simulink model "s_VI_Operational_pd_wG_ctrl_14bb"  (Simulink 8.4)
settings: Solver=ode45  SolverMode=SingleTasking  StartTime=0.0  StopTime=10.0  RelTol=1e-3
values from neighbouring files (symbols this model uses):
  Kd = 50    [m_IV_run_pd_wG_control_operational.m]
  Kp = 2500    [m_IV_run_pd_wG_control_operational.m]
settings Model: Creator=a_bad  LastModifiedBy=a_bad  CovMetricSettings=dwe  CovHtmlReporting=off  covSaveCumulativeToWorkspaceVar=off  CovSaveSingleToWorkspaceVar=off  CovExternalEMLEnable=on  CovSFcnEnable=on
settings DataIOCC: LimitDataPoints=off  SaveFormat=StructureWithTime  SignalLoggingSaveFormat=Dataset
settings OptimizationCC: ExpressionDepthLimit=128
settings DebuggingCC: AlgebraicLoopMsg=none  UnderspecifiedInitializationDetection=Simplified  MergeDetectMultiDrivingBlocksExec=error  SolverPrmCheckMsg=none  FcnCallInpInsideContextMsg=EnableAllAsError  FrameProcessingCompatibilityMsg=error  StateNameClashWarn=none  SFUnexpectedBacktrackingDiag=error  SFNoUnconditionalDefaultTransitionDiag=error
settings HardwareCC: ProdBitPerPointer=64  ProdLargestAtomicFloat=Float  ProdIntDivRoundTo=Zero  ProdEndianess=LittleEndian  ProdHWDeviceType=Specified
settings ModelReferenceCC: PropagateSignalLabelsOutOfModel=on
settings GRTTargetCC: TargetLangStandard=C99 (ISO)  GeneratePreprocessorConditionals=Use local settings  CombineOutputUpdateFcns=on  GRTInterface=off

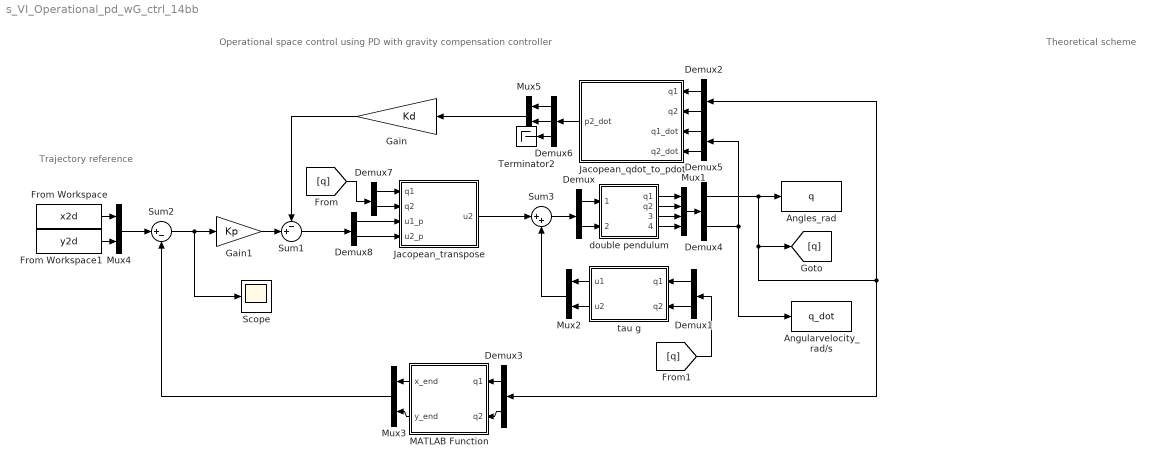
== system s_VI_Operational_pd_wG_ctrl_14bb ==
  note: Theoretical scheme
  note: Trajectory
      | reference
  note: Operational space control using PD with gravity compensation controller
  Angles_rad : ToWorkspace  VariableName=q  SaveFormat=Timeseries  SampleTime=-1
  Angularvelocity_rad/s : ToWorkspace  VariableName=q_dot  SaveFormat=Timeseries  SampleTime=-1
  Demux{,1..5,7..8} (8 alike) : Demux  Outputs=2
  Demux6 : Demux  Outputs=3
  From Workspace : FromWorkspace  VariableName=x2d  SampleTime=0
  From Workspace1 : FromWorkspace  VariableName=y2d  SampleTime=0
  Gain : Gain  Gain=Kd
  Gain1 : Gain  Gain=Kp
  Jacopean_qdot_to_pdot : MATLAB Function  TreatAsAtomicUnit=on
      settings: PermitHierarchicalResolution=ParametersOnly
  Jacopean_transpose : MATLAB Function  TreatAsAtomicUnit=on
      settings: PermitHierarchicalResolution=ParametersOnly
  MATLAB Function : MATLAB Function  TreatAsAtomicUnit=on
      settings: PermitHierarchicalResolution=ParametersOnly
  Mux1 : Mux
  Mux{2..5} (4 alike) : Mux  Inputs=2
  Scope : Scope
      settings: TimeRange=auto  MaxDataPoints=5000  SaveToWorkspace=off  SaveName=ScopeData  YMin=-0.05308  YMax=0.10902  SampleTime=-1
  Sum1 : Sum  Inputs=-+|
  Sum2 : Sum  Inputs=|+-
  Sum3 : Sum  Inputs=|++
  Terminator2 : Terminator
  "double pendulum " : Subsystem
      mask Display: image('294px-Double-Pendulum.svg.png');
  "tau g " : MATLAB Function  TreatAsAtomicUnit=on
      settings: PermitHierarchicalResolution=ParametersOnly
  wires:
  "double pendulum "/1(q1) -> Mux1/1
  Demux/1 -> "double pendulum "/1(Tau1)
  Demux/2 -> "double pendulum "/2("Tau2 ")
  "double pendulum "/4(q2_dot) -> Mux1/4
  "double pendulum "/2("q2  ") -> Mux1/2
  "double pendulum "/3("q1_dot ") -> Mux1/3
  Mux1/1 -> Demux4/1
  Demux4/2 -> Angularvelocity_rad/s/1, Demux5/1
  Demux4/1 -> Demux3/1, Demux2/1, [q], Angles_rad/1
  From Workspace/1 -> Mux4/1
  From Workspace1/1 -> Mux4/2
  Mux4/1 -> Sum2/1
  Demux1/1 -> "tau g "/1(q1)
  Demux1/2 -> "tau g "/2(q2)
  "tau g "/1(u1) -> Mux2/1
  "tau g "/2(u2) -> Mux2/2
  Sum3/1 -> Demux/1
  Demux3/1 -> MATLAB Function/1(q1)
  Demux3/2 -> MATLAB Function/2(q2)
  Mux2/1 -> Sum3/2
  MATLAB Function/1(x_end) -> Mux3/1
  MATLAB Function/2(y_end) -> Mux3/2
  Mux3/1 -> Sum2/2
  Demux2/1 -> Jacopean_qdot_to_pdot/1(q1)
  Demux2/2 -> Jacopean_qdot_to_pdot/2(q2)
  Demux5/1 -> Jacopean_qdot_to_pdot/3(q1_dot)
  Demux5/2 -> Jacopean_qdot_to_pdot/4(q2_dot)
  Jacopean_qdot_to_pdot/1(p2_dot) -> Demux6/1
  Demux6/3 -> Terminator2/1
  Demux6/1 -> Mux5/1
  Demux6/2 -> Mux5/2
  Mux5/1 -> Gain/1
  Sum2/1 -> Scope/1, Gain1/1
  Gain/1 -> Sum1/1
  Gain1/1 -> Sum1/2
  Demux7/1 -> Jacopean_transpose/1(q1)
  Demux7/2 -> Jacopean_transpose/2(q2)
  [q] -> Demux7/1
  Sum1/1 -> Demux8/1
  Demux8/1 -> Jacopean_transpose/3(u1_p)
  Demux8/2 -> Jacopean_transpose/4(u2_p)
  Jacopean_transpose/1(u2) -> Sum3/1
  [q] -> Demux1/1

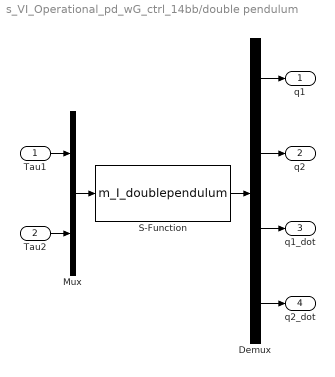
== system s_VI_Operational_pd_wG_ctrl_14bb/double pendulum  ==
  Tau1 : Inport
  "Tau2 " : Inport  Port=2
  Demux : Demux
  Mux : Mux  Inputs=2
  S-Function : S-Function  FunctionName=m_I_doublependulum  Parameters=pi/2 -pi 0 0  SFunctionDeploymentMode=off  EnableBusSupport=off
  q1 : Outport
  "q2  " : Outport  Port=2
  "q1_dot " : Outport  Port=3
  q2_dot : Outport  Port=4
  wires:
  Mux/1 -> S-Function/1
  S-Function/1 -> Demux/1
  Tau1/1 -> Mux/1
  "Tau2 "/1 -> Mux/2
  Demux/4 -> q2_dot/1
  Demux/3 -> "q1_dot "/1
  Demux/2 -> "q2  "/1
  Demux/1 -> q1/1

== matlab function tau g  ==
  data: q1 input double; u1 output double; q2 input double; u2 output double
function [u1,u2] = fcn(q1,q2)
Grav=10;     %%Gravity acceleration constant
M=1;       
L1=1;
L2=1;
Gz=1;
beta=20;
G1=M*(L1^2+L2^2)+Gz; G2=M*L2^2+Gz;
g1=M*Grav*(L1*cos(q1)+L2*cos(q1+q2));    g2=M*Grav*L2*cos(q1+q2);
u1=g1;u2=g2;

== matlab function MATLAB Function ==
  data: q1 input double; x_end output double; q2 input double; y_end output double
function [x_end,y_end] = fcn(q1,q2)

L1=1;L2=1;

x = [L1*cos(q1),  L1*cos(q1)+L2*cos(q1+q2)];
y = [L1*sin(q1),  L1*sin(q1)+L2*sin(q1+q2)];
x_end=x(2);
y_end=y(2);

== matlab function Jacopean_qdot_to_pdot ==
  data: q1 input double; q2 input double; q1_dot input double; q2_dot input double; p2_dot output double
function p2_dot  = fcn(q1,q2,q1_dot,q2_dot)

L1=1;L2=1;
A=[-L1*sin(q1)           0;
    L1*cos(q1)           0;
    1                    0];
B=[-L1*sin(q1)-L2*sin(q1+q2)        -L2*sin(q1+q2);
    L1*cos(q1)+L2*cos(q1+q2)         L2*cos(q1+q2);
    1                                1              ];
p1_dot=A*[q1_dot;q2_dot];
p2_dot=B*[q1_dot;q2_dot];

== matlab function Jacopean_transpose ==
  data: q1 input double; q2 input double; u1_p input double; u2_p input double; u2 output double
function u2  = fcn(q1,q2,u1_p,u2_p)

L1=1;L2=1;
A=[-L1*sin(q1)           0;
    L1*cos(q1)           0;
  ];

B=[-L1*sin(q1)-L2*sin(q1+q2)        -L2*sin(q1+q2);
    L1*cos(q1)+L2*cos(q1+q2)         L2*cos(q1+q2);
   ];

u1=A'*[u1_p;u2_p];
u2=B'*[u1_p;u2_p];
